simulink library "mpc555extras"  (Simulink 6.0)
settings: Solver=ode45  SolverMode=SingleTasking  StartTime=0.0  StopTime=10.0  RelTol=1e-3
undefined symbols (not defined in the file or in its folder): INT_LEVEL6
libraries: mpc555extras x13, driver_interface_library x7, simulink x4, mpc555interrupts x1
settings Model: Creator=The MathWorks Inc.  LastModifiedBy=batserve  ExtModeAutoUpdateStatusClock=off
settings DataIOCC: SignalLoggingName=logsOut
settings OptimizationCC: BooleanDataType=off
settings DebuggingCC: CheckExecutionContextPreStartOutputMsg=on  CheckExecutionContextRuntimeOutputMsg=on  SolverPrmCheckMsg=none
settings HardwareCC: TargetUnknown=on
settings ModelReferenceCC: UpdateModelReferenceTargets=IfOutOfDate

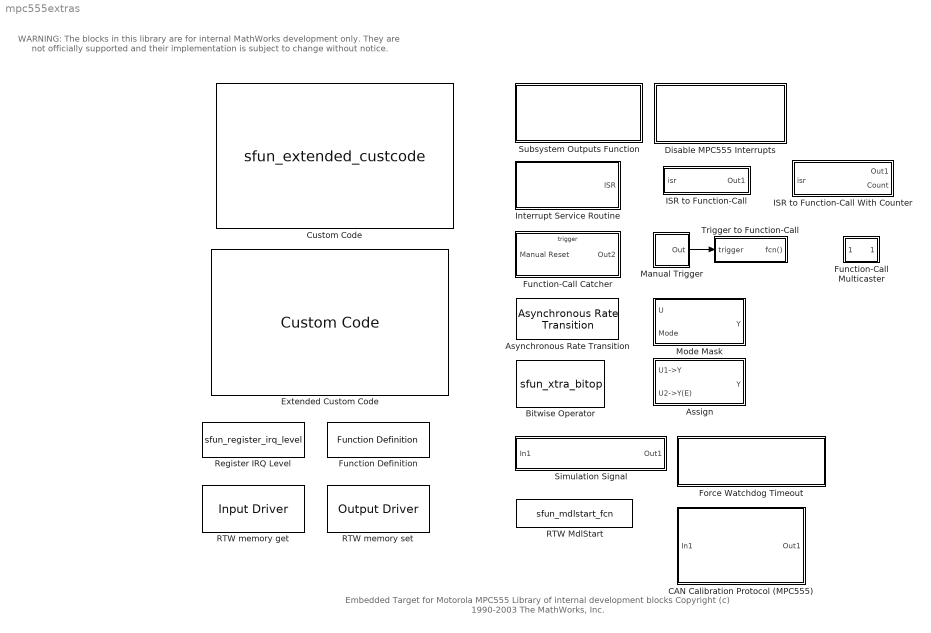
== system mpc555extras ==
  note: WARNING:
      | The blocks in this library are for internal MathWorks development only.
      | They are not officially supported and their implementation is subject to change without notice.
  note: Embedded Target for Motorola MPC555
      | Library of internal development blocks
      | Copyright (c) 1990-2003 The MathWorks, Inc.
  Assign : Subsystem  PropExecContextAcrossSSBoundary=on  mask(Assignment Block){width=5, elements=[2 3]}
      mask prompts: width "Input Width"
      mask help: Replace the specified elements in the input vector with elements from the second vector. You must specify the width of the input signal exactly.
      mask init:
      | elements_split = setdiff([1:width],elements);
      | [s,idx] = sort( [ elements_split elements]);
      | elements_merge = idx;
  Asynchronous Rate Transition : mpc555interrupts/Asynchronous Rate Transition  sample_time=-1
  Bitwise Operator : S-Function  FunctionName=sfun_xtra_bitop  Parameters=UseBitMask,NumInputPorts,BitMask,logicop,zeroTest  mask(Fixed-Point Bitwise Operator){logicop=AND, zeroTest=No Test, UseBitMask=on, NumInputPorts=1, BitMask=bin2dec('11011001'), maskInBinary=off}
      mask prompts: logicop "Operator:"; zeroTest "Zero Test"; UseBitMask "Use bit mask ..."; NumInputPorts "Number of input ports:"; BitMask "Bit Mask"; maskInBinary "Show Mask As Binary"
      mask help: Perform the specified bitwise operation on the inputs. The output data type should represent zero exactly.
      mask init:
      | [BitMask, str ] = sfun_bitop_msk('init',UseBitMask,NumInputPorts,BitMask,logicop,zeroTest);
      mask Help: web(fpbhelp('bitwiseoperator'));
      mask StyleString: popup(AND|OR|NAND|NOR|XOR|NOT|SHIFT LEFT|SHIFT RIGHT|BIT SET|BIT CLEAR|NOT a AND b|a AND NOT b|NOT a OR b|a OR NOT b ),popup(No Test|Test  If Zero|Test If Not Zero),checkbox,edit,edit,checkbox
      mask CallbackString: sfun_bitop_msk('callback')||sfun_bitop_msk('callback')|||
      mask Display: fprintf(['Bitwise\n',str])
  CAN Calibration Protocol (MPC555) : Subsystem  PropExecContextAcrossSSBoundary=on
      mask init:
      | block = 'mpc555drivers/CAN 2.0B Controller Module/CAN Calibration Protocol';                                                                 
      |                                                                           
      | load_system(strtok(block, '/'));                                           
      |                                                                           
      | regexprep(block, '\s',' ');                                                
      | msg = sprintf('Please replace the CCP block with the updated version: "%s" ', block);                             
      | error(msg);
      mask Display: disp(sprintf('Please update\nthe model\nfor a link\nto a\nreplacement block'));
  Custom Code : S-Function  FunctionName=sfun_extended_custcode  mask(Subsystem Custom Coder){unique=Generate for every instance, key='', location=Subsystem Enable Function, top='/* Top Code */', middle='/*Middle Code */', bottom='/*Bottom Code*/'}
      mask prompts: unique "Unique Code Code Generation"
      mask init:
      | [ dispstr,rtwdata ] = mask_custom_code(unique,key,location,top,middle,bottom);
      | set_param(gcb,'rtwdata',rtwdata);
      settings: AttributesFormatString=\n\n
      mask StyleString: popup(Generate for every instance|Generate once per functional mask|Model Singleton),edit,popup(Header File|Parameter File|Source File|Registration File|Subsystem Start Function|Subsystem Initialize Function|Subsystem Terminate Function|Subsystem Enable Function|Subsystem Disable Function|Subsystem Outputs Function|Subsystem Update Function|Subsystem Derivatives Function|Registration Function|Model Start Function|Model Initialize Function|Model Terminate Function|Model Outputs Function|Model Update Function|Model Derivatives Function),edit,edit,edit
      mask Display: text(0.1,0.5,dispstr,'horizontalAlignment','left')
  Disable MPC555 Interrupts : Subsystem  Tag=Disable MPC555 Interrupts  PropExecContextAcrossSSBoundary=on  mask(Disable MPC555 Interrupts){}
      mask help:
      | Disable MPC555 Interrupts during the model outputs function.
      |
      | Be carefull using this block as it may block a faster rate task from executing in time. Use it only in atomic subsystems that may be accessing hardware resources that need protection against interrupt access.
      mask init:
      | [top,bottom,dispstr] = mpc555_disable_interrupts('getcode',gcb);
      mask Display: disp(dispstr)
  Extended Custom Code : driver_interface_library/Custom Code
  Force Watchdog Timeout : Subsystem  TreatAsAtomicUnit=on  PropExecContextAcrossSSBoundary=on  mask(Processor Reset){}
      mask help:
      | As soon as this block executes interrupts are disabled and the processor enters an infinite loop. The watchdog timer will then time out and reset the processor.
      |
      | This block mus be placed in an action subsystem such as an if, then, else subsystem or a function call subsystem.
      mask init:
      | read_tunable_parameters;
      mask Help:
      | As soon as this block executes interrupts are disabled and the processor enters an infinite loop. The watchdog timer will then time out and reset the processor.<p>
      | 
      | This block mus be placed in an action subsystem such as an if, then, else subsystem or a function call subsystem.
      mask Display: disp('Processor Reset\nForce Watchdog Timeout');
  Function Definition : driver_interface_library/Function Definition  function_name='void func(void)'
  Function-Call Multicaster : Subsystem  PropExecContextAcrossSSBoundary=on
      mask Type: Function Call Multicaster
      mask Description: The input to this block should be a function call. The output of the block can be demuxed so that multiple function call subsystems can be triggered off the same function call.
      mask Display:
      | plot([0 2],[0.5 0.5]);
      | plot([0.5 1],[0.6 0.6]);
      | plot([0.5 1],[0.4 0.4]);
      | plot([0.8 1],[0.7 0.7]);
      | plot([0.8 1],[0.3 0.3]);
      | 
      | plot([1 1],[0.3 0.7])
      | plot([0.95 0.95],[0.2 0.8])
      | plot([0.9 0.9],[0.2 0.8])
  Function-Call Catcher : Subsystem  TreatAsAtomicUnit=on  PropExecContextAcrossSSBoundary=on
      mask Type: Function Call Catcher
      mask Description: Feed in multiple function call trigger via a mux into the top. The block wait till every function trigger has fired at least once before firing it's output trigger then reseting it's counters
  ISR to Function-Call : Subsystem  PropExecContextAcrossSSBoundary=on  mask{t=1}
      mask prompts: t "Sample Period"
      mask help: Converts an interrupt service routine call to a "if action" call at a specified sample rate.
      settings: AttributesFormatString=sample time = %<t>
      mask Display:
      | plot([0.2 0.4 0.5 0.6 0.7 0.75 ],[0.5 0.5 0.7 0.3 0.5 0.5])
      | plot([0.2 0.4 0.5 0.6 0.7 0.75 ],1-[0.5 0.5 0.7 0.3 0.5 0.5])
      | plot([0.2 0.4 0.5 0.6 0.7 0.75 ],1- [0.5 0.5 0.7 0.3 0.5 0.5]+0.1)
      | port_label('input',1,'isr')
      | port_label('output',1,'if { }')
  ISR to Function-Call With Counter : Subsystem  PropExecContextAcrossSSBoundary=on  mask{t=1}
      mask prompts: t "Sample Period"
      mask help: Converts an interrupt service routine call to a "if action" call at a specified sample rate. It also has an output that provides the number of times the interrupt has executed since it was last polled.
      settings: AttributesFormatString=sample time = %<t>
      mask Display:
      | plot([0.2 0.4 0.5 0.6 0.7 0.75 ],[0.5 0.5 0.7 0.3 0.5 0.5])
      | plot([0.2 0.4 0.5 0.6 0.7 0.75 ],1-[0.5 0.5 0.7 0.3 0.5 0.5])
      | plot([0.2 0.4 0.5 0.6 0.7 0.75 ],1- [0.5 0.5 0.7 0.3 0.5 0.5]+0.1)
      | port_label('input',1,'isr')
      | port_label('output',1,'if { }')
      | port_label('output',2,'count')
  Interrupt Service Routine : Subsystem  PropExecContextAcrossSSBoundary=on  mask{callback=EXT_IRQ0, float_flag=Yes}
      mask prompts: callback "ISR Source"; float_flag "Uses Floating Point?"
      mask help: Choose the interrupt source for your ISR generator. For faster interrupts you can choose not to support floating point. However if you choose not to support floating point in the system and you place blocks in the system that do you floating point operation then the program will throw a floating point exception at run-time.
      mask init:
      | [f_proto,dispstr,reg_callback ]  = mask_isr_callback(gcbh,callback,float_flag);
      mask StyleString: popup(EXT_IRQ0|INT_LEVEL0|EXT_IRQ1|INT_LEVEL1|EXT_IRQ2|INT_LEVEL2|EXT_IRQ3|INT_LEVEL3|EXT_IRQ4|INT_LEVEL4|EXT_IRQ5|INT_LEVEL5|EXT_IRQ6|INT_LEVEL6|EXT_IRQ7|INT_LEVEL7|INT_LEVEL8|INT_LEVEL9|INT_LEVEL10|INT_LEVEL11|INT_LEVEL12|INT_LEVEL13|INT_LEVEL14|INT_LEVEL15|INT_LEVEL16|INT_LEVEL17|INT_LEVEL18|INT_LEVEL19|INT_LEVEL20|INT_LEVEL21|INT_LEVEL22|INT_LEVEL23|INT_LEVEL24|INT_LEVEL25|INT_LEVEL26|INT_LEVEL27|INT_LEVEL28|INT_LEVEL29|INT_LEVEL30|INT_LEVEL31),popup(Yes|No)
      mask Display: disp(dispstr)
  Manual Trigger : Subsystem  PropExecContextAcrossSSBoundary=on  mask(Manual Trigger){value=-1}
      mask prompts: value "Output value:"
      mask init:
      | if (value==1)
      |   dispStr = 'HIGH';
      | else % (value == -1)
      |   dispStr = 'LOW';
      | end
      settings: OpenFcn=oldValue = str2num(get_param(gcb, 'value')); if (oldValue==1), set_param(gcb, 'value', '-1'); else, set_param(gcb, 'value', '1'); end
      mask Display: disp(dispStr)
  Mode Mask : Subsystem  PropExecContextAcrossSSBoundary=on  mask(Mode based mask){width=5, elements=[2 3], mode_inputs=[1 2], mode_outputs=[0 0]}
      mask prompts: width "Input Width"; elements "Mode Elements"; mode_inputs "Mode Inputs"; mode_outputs "Mode Outputs"
      mask help: Enables selective switching of input elements based on a single scalar mode value.
      mask Help:
      | <ul>
      | <li>Specify the input width exactly.
      | <li>The mode elements are the elements of the input
      | vector that can be switched. Specify their indicies
      | <li> The mode inputs are the mode values for each input
      | that when the mode input equals the value the input element
      | will be switched
      | <li> The mode outputs are the alternative values for each element that is switched in if it's mode value is equal.
      | </ul>
  RTW MdlStart : S-Function  FunctionName=sfun_mdlstart_fcn
      mask Type: RTW MdlStart Function
      mask Description:
      | Forces downstream triggered blocks to run at mdlStart.
      | 
      | Be carefull with this block. You should not put in the triggered subsystem any blocks
      | which have state. This block is primarily to be used to perform device driver initialization.
      | 
      | The blocks in the downstream triggered subsystem will not run during simulation
      | or Simulink Accelerator.
      mask Display: disp('RTW MdlStart Function')
  RTW memory get : driver_interface_library/Input Driver  t=1  expr='MIOS1[%<i>][%<p>]'  portWidth=6  pOpt=[2 3 6 8 3 9]  expression_type=Not expression
  RTW memory set : driver_interface_library/Output Driver  operation_type=LHS Assignment  input_is_contiguous=off  t=-1  expr='*Y_ADDR'  port_width=1  pOpt=[]
  Register IRQ Level : S-Function  FunctionName=sfun_register_irq_level  Parameters=irqLevel  mask{irqLevel=INT_LEVEL6}
      mask prompts: irqLevel "IRQ Level"
      mask Display: disp('Register IRQ level')
  Simulation Signal : Subsystem  PropExecContextAcrossSSBoundary=on  mask(Simulation-only signal){baseName=SimSignal}
      mask prompts: baseName "Base name for signal identifier:"
      mask help: Only produce an identifier for this signal when generating code for use in simulation (e.g., Accelerator, Processor-in-the-loop and S-Function targets).
      mask init:
      | InportBlock = [gcb, '/In1'];
      | hPorts = get_param(InportBlock, 'PortHandles');
      | hPort = hPorts.Outport;
      | signalName = getuniquesignalname(hPort, baseName);
      | eval([signalName, '=SimOnly.Signal;']);
      | set_param(hPort, 'Name', signalName);
      mask Display: disp(['SimOnlySignal: ', signalName])
  Subsystem Outputs Function : Subsystem  PropExecContextAcrossSSBoundary=on
      settings: OpenFcn=ccopenfcn('Subsystem Outputs Function')
      mask Type: Subsystem Outputs Function
      mask Description: Place this block in an atomic subsystem to ensure that the subsystem is protected from interrupts during the model outputs function. This block should not be used recursively.
      mask Display: disp('Disable Interrupts \nIn Outputs Function Of\nAtomic Subsytem');
  Trigger to Function-Call : Subsystem  PropExecContextAcrossSSBoundary=on
      mask Type: Trigger to function call conversion
      mask Description: Converts a Simulink trigger signal to a function call trigger signal.
  wires:
  Manual Trigger/1(Out) -> Trigger to Function-Call/1(trigger)

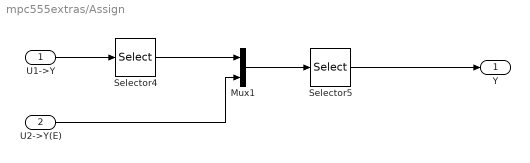
== system mpc555extras/Assign ==
  U1->Y : Inport  Port=1  LatchInput=off
  U2->Y(E) : Inport  Port=2  LatchInput=off
  Mux1 : Mux  Inputs=2
  Selector4 : Selector  Elements=elements_split  InputPortWidth=width
  Selector5 : Selector  Elements=elements_merge  InputPortWidth=width
  Y : Outport
  wires:
  Selector4/1 -> Mux1/1
  Mux1/1 -> Selector5/1
  U1->Y/1 -> Selector4/1
  Selector5/1 -> Y/1
  U2->Y(E)/1 -> Mux1/2

== system mpc555extras/CAN Calibration Protocol (MPC555) ==
  In1 : Inport  Port=1  LatchInput=off
  Out1 : Outport
  wires:
  In1/1 -> Out1/1

== system mpc555extras/Disable MPC555 Interrupts ==
  Disable MPC555 Interrupts : mpc555extras/Custom Code  Tag=Disable MPC555 Interrupts  unique=Generate for every instance  key=''  location=Subsystem Outputs Function  top=top  middle=''  bottom=bottom

== system mpc555extras/Force Watchdog Timeout ==
  Constant : Constant
  Force Watchdog Timeout : mpc555extras/Custom Code  unique=Generate for every instance  key=''  location=Subsystem Outputs Function  top=''  middle=''  bottom='EID(); for(;;);'
  Terminator : Terminator
  wires:
  Constant/1 -> Terminator/1

== system mpc555extras/Function-Call Multicaster ==
  fcn_in : Inport  Port=1  LatchInput=off
  Subsystem : Subsystem  TreatAsAtomicUnit=on  PropExecContextAcrossSSBoundary=on
  fcn1 : Outport
  wires:
  Subsystem/1(Out1) -> fcn1/1
  fcn_in/1 -> Subsystem/Trigger

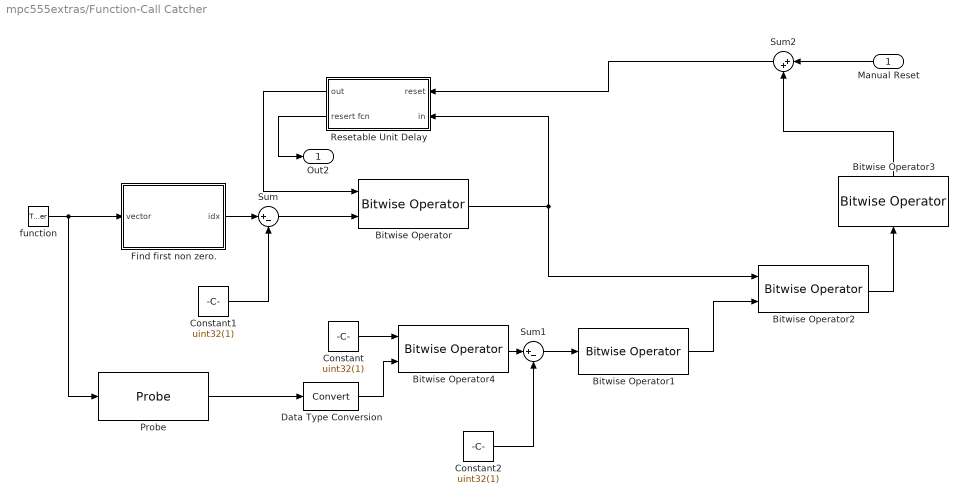
== system mpc555extras/Function-Call Catcher ==
  Manual Reset : Inport  Orientation=left  Port=1  LatchInput=off
  function : TriggerPort  TriggerType=function-call  StatesWhenEnabling=reset  ShowOutputPort=on  OutputDataType=int8  ZeroCross=off
  Bitwise Operator : mpc555extras/Bitwise Operator  logicop=BIT SET  zeroTest=No Test  UseBitMask=off  NumInputPorts=2  BitMask=bin2dec('11011001')  maskInBinary=off
  Bitwise Operator1 : mpc555extras/Bitwise Operator  logicop=NOT  zeroTest=No Test  UseBitMask=on  BitMask=bin2dec('11011001')  maskInBinary=off
  Bitwise Operator2 : mpc555extras/Bitwise Operator  logicop=OR  zeroTest=No Test  UseBitMask=off  NumInputPorts=2  BitMask=bin2dec('11011001')  maskInBinary=off
  Bitwise Operator3 : mpc555extras/Bitwise Operator  Orientation=up  logicop=NOT  zeroTest="Test  If Zero"  UseBitMask=on  BitMask=bin2dec('11011001')  maskInBinary=off
  Bitwise Operator4 : mpc555extras/Bitwise Operator  logicop=SHIFT LEFT  zeroTest=No Test  UseBitMask=off  NumInputPorts=2  BitMask=bin2dec('11011001')  maskInBinary=off
  Constant : Constant  Value=uint32(1)
  Constant1 : Constant  Value=uint32(1)
  Constant2 : Constant  Value=uint32(1)
  Data Type Conversion : DataTypeConversion  OutDataTypeMode=uint32  RndMeth=Zero
  Find first non zero. : Subsystem  PropExecContextAcrossSSBoundary=on
  Probe : Probe  ProbeSampleTime=off  ProbeComplexSignal=off
  Resetable Unit Delay : Subsystem  Orientation=left  PropExecContextAcrossSSBoundary=on  mask(Resetable Unit Delay){reset=uint32(0), t=-1}
      mask prompts: reset "Initial State"; t "Sample Time"
  Sum : Sum  Inputs=|+-  InputSameDT=on
  Sum1 : Sum  Inputs=|+-  InputSameDT=on
  Sum2 : Sum  Orientation=left  Inputs=|++  SaturateOnIntegerOverflow=on  InputSameDT=on
  Out2 : Outport
  wires:
  Sum2/1 -> Resetable Unit Delay/1(reset)
  Bitwise Operator3/1 -> Sum2/2
  Manual Reset/1 -> Sum2/1
  Constant2/1 -> Sum1/2
  Sum1/1 -> Bitwise Operator1/1
  Bitwise Operator4/1 -> Sum1/1
  Constant/1 -> Bitwise Operator4/1
  Bitwise Operator2/1 -> Bitwise Operator3/1
  Bitwise Operator1/1 -> Bitwise Operator2/2
  Resetable Unit Delay/1(out) -> Bitwise Operator/1
  Bitwise Operator/1 -> Bitwise Operator2/1, Resetable Unit Delay/2(in)
  function/1 -> Probe/1, Find first non zero./1(vector)
  Find first non zero./1(idx) -> Sum/1
  Sum/1 -> Bitwise Operator/2
  Constant1/1 -> Sum/2
  Resetable Unit Delay/2(resert fcn) -> Out2/1
  Data Type Conversion/1 -> Bitwise Operator4/2
  Probe/1 -> Data Type Conversion/1

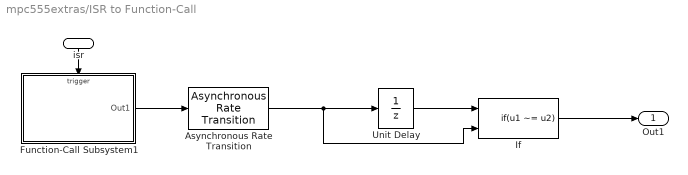
== system mpc555extras/ISR to Function-Call ==
  isr : Inport  Orientation=down  Port=1  LatchInput=off
  Asynchronous Rate Transition : mpc555extras/Asynchronous Rate Transition  sample_time=-1
  Function-Call Subsystem1 : Subsystem  TreatAsAtomicUnit=on  PropExecContextAcrossSSBoundary=on
  If : If  NumInputs=2  IfExpression=u1 ~= u2  ShowElse=off  ZeroCross=off
  Unit Delay : UnitDelay  SampleTime=t
  Out1 : Outport
  wires:
  Function-Call Subsystem1/1(Out1) -> Asynchronous Rate Transition/1
  Asynchronous Rate Transition/1 -> If/2, Unit Delay/1
  isr/1 -> Function-Call Subsystem1/Trigger
  If/1 -> Out1/1
  Unit Delay/1 -> If/1

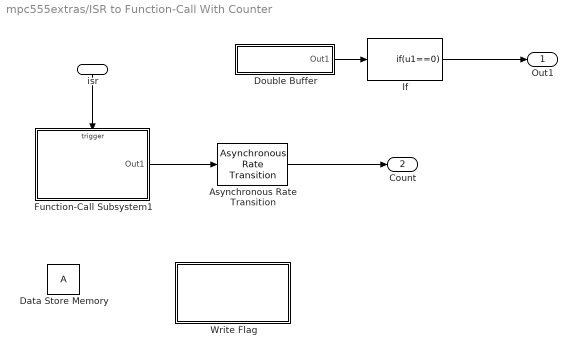
== system mpc555extras/ISR to Function-Call With Counter ==
  isr : Inport  Orientation=down  Port=1  LatchInput=off
  Asynchronous Rate Transition : mpc555extras/Asynchronous Rate Transition  sample_time=t
  Data Store Memory : DataStoreMemory  DialogController=Simulink.DDGSource  DataStoreName=A  InitialValue=1
  Double Buffer : Subsystem  TreatAsAtomicUnit=on  PropExecContextAcrossSSBoundary=on
  Function-Call Subsystem1 : Subsystem  TreatAsAtomicUnit=on  PropExecContextAcrossSSBoundary=on
  If : If  IfExpression=u1==0  ShowElse=off  ZeroCross=off
  Write Flag : Subsystem  TreatAsAtomicUnit=on  PropExecContextAcrossSSBoundary=on
  Out1 : Outport
  Count : Outport  Port=2
  wires:
  Double Buffer/1(Out1) -> If/1
  Asynchronous Rate Transition/1 -> Count/1
  If/1 -> Out1/1
  isr/1 -> Function-Call Subsystem1/Trigger
  Function-Call Subsystem1/1(Out1) -> Asynchronous Rate Transition/1

== system mpc555extras/Interrupt Service Routine ==
  Custom Code : mpc555extras/Custom Code  unique=Generate for every instance  key=''  location=Model Start Function  top=reg_callback  middle=''  bottom=''
  Function Definition : driver_interface_library/Function Definition  function_name=f_proto
  Header File : Subsystem  Tag=line1 line2  PropExecContextAcrossSSBoundary=on
      settings: CopyFcn=cccopyfcn(gcb)  OpenFcn=ccopenfcn('Header File')
      mask Type: Header File
      mask Description: Add code to model .h file
      mask Help: This header file block contains text fields to insert custom user code at the top and bottom of model.h file.
      mask Display: disp('Header\nFile');
  ISR : Outport
  wires:
  Function Definition/1 -> ISR/1

== system mpc555extras/Manual Trigger ==
  Output value : Constant  Value=value
  Out : Outport
  wires:
  Output value/1 -> Out/1

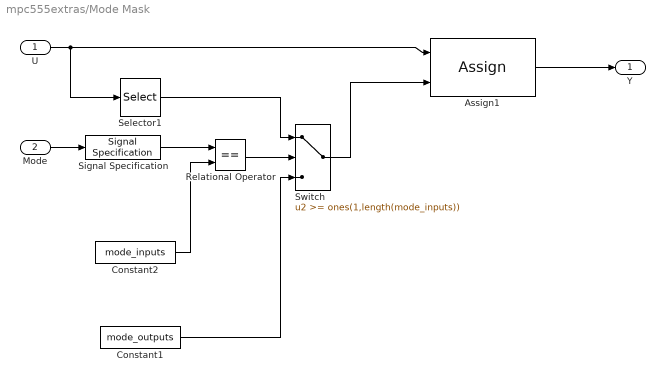
== system mpc555extras/Mode Mask ==
  U : Inport  Port=1  LatchInput=off
  Mode : Inport  Port=2  LatchInput=off
  Assign1 : mpc555extras/Assign  width=width  elements=elements
  Constant1 : Constant  Value=mode_outputs
  Constant2 : Constant  Value=mode_inputs
  Relational Operator : RelationalOperator  Operator===  InputSameDT=on
  Selector1 : Selector  Elements=elements  InputPortWidth=width
  Signal Specification : simulink/Signal Attributes/Signal Specification  D=1  Ts=-1  DataType=auto  OutDataType=sfix(16)  OutScaling=2^0
      settings: SignalType=auto  SamplingMode=auto
  Switch : Switch  Threshold=ones(1,length(mode_inputs))  InputSameDT=on
  Y : Outport
  wires:
  Constant2/1 -> Relational Operator/2
  Relational Operator/1 -> Switch/2
  U/1 -> Assign1/1, Selector1/1
  Constant1/1 -> Switch/3
  Selector1/1 -> Switch/1
  Switch/1 -> Assign1/2
  Assign1/1 -> Y/1
  Mode/1 -> Signal Specification/1
  Signal Specification/1 -> Relational Operator/1

== system mpc555extras/Simulation Signal ==
  In1 : Inport  Port=1  LatchInput=off
  Out1 : Outport
  wires:
  In1/1 -> Out1/1  "SimSignal1"

== system mpc555extras/Subsystem Outputs Function ==

== system mpc555extras/Trigger to Function-Call ==
  trigger : Inport  Orientation=down  Port=1  LatchInput=off
  trigger2fcn : Subsystem  TreatAsAtomicUnit=on  PropExecContextAcrossSSBoundary=on
  fcn() : Outport
  wires:
  trigger2fcn/1(fcn()) -> fcn()/1
  trigger/1 -> trigger2fcn/Trigger

== system mpc555extras/Function-Call Multicaster/Subsystem ==
  Trigger : TriggerPort  TriggerType=function-call  StatesWhenEnabling=reset  ZeroCross=off
  Function-Call Generator : simulink/Ports & Subsystems/Function-Call Generator  sample_time=-1  numberOfIterations=1
  Out1 : Outport
  wires:
  Function-Call Generator/1 -> Out1/1

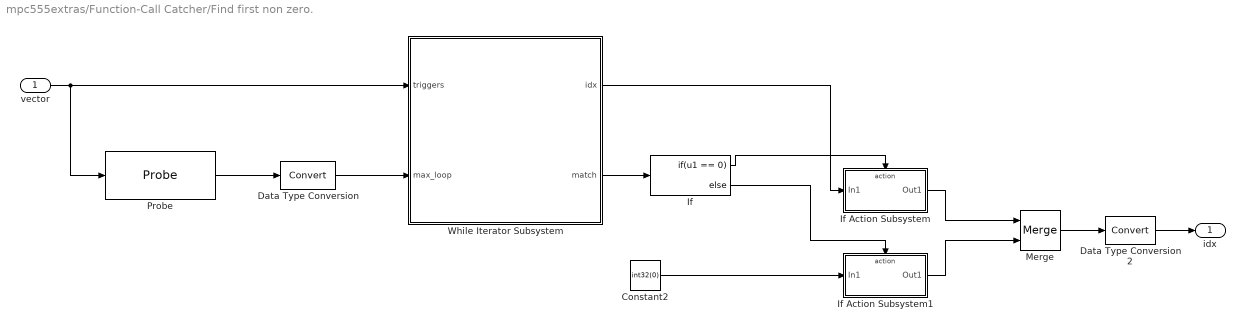
== system mpc555extras/Function-Call Catcher/Find first non zero. ==
  vector : Inport  Port=1  LatchInput=off
  Constant2 : Constant  Value=int32(0)
  Data Type Conversion : DataTypeConversion  OutDataTypeMode=int32  RndMeth=Zero
  Data Type Conversion2 : DataTypeConversion  OutDataTypeMode=uint32  RndMeth=Zero
  If : If  IfExpression=u1 == 0  ZeroCross=off
  If Action Subsystem : Subsystem  TreatAsAtomicUnit=on  PropExecContextAcrossSSBoundary=on
  If Action Subsystem1 : Subsystem  TreatAsAtomicUnit=on  PropExecContextAcrossSSBoundary=on
  Merge : Merge
  Probe : Probe  ProbeSampleTime=off  ProbeComplexSignal=off
  While Iterator Subsystem : Subsystem  TreatAsAtomicUnit=on  PropExecContextAcrossSSBoundary=on
  idx : Outport
  wires:
  Data Type Conversion/1 -> While Iterator Subsystem/2(max_loop)
  Merge/1 -> Data Type Conversion2/1
  If Action Subsystem1/1(Out1) -> Merge/2
  If Action Subsystem/1(Out1) -> Merge/1
  If/2 -> If Action Subsystem1/Action
  If/1 -> If Action Subsystem/Action
  Constant2/1 -> If Action Subsystem1/1(In1)
  While Iterator Subsystem/2(match) -> If/1
  While Iterator Subsystem/1(idx) -> If Action Subsystem/1(In1)
  Probe/1 -> Data Type Conversion/1
  vector/1 -> While Iterator Subsystem/1(triggers), Probe/1
  Data Type Conversion2/1 -> idx/1

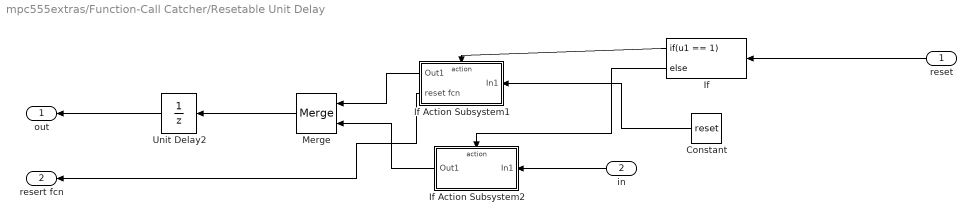
== system mpc555extras/Function-Call Catcher/Resetable Unit Delay ==
  reset : Inport  Orientation=left  Port=1  LatchInput=off
  in : Inport  Orientation=left  Port=2  LatchInput=off
  Constant : Constant  Orientation=left  Value=reset
  If : If  Orientation=left  IfExpression=u1 == 1  ZeroCross=off
  If Action Subsystem1 : Subsystem  Orientation=left  TreatAsAtomicUnit=on  PropExecContextAcrossSSBoundary=on
  If Action Subsystem2 : Subsystem  Orientation=left  TreatAsAtomicUnit=on  PropExecContextAcrossSSBoundary=on
  Merge : Merge  Orientation=left
  Unit Delay2 : UnitDelay  Orientation=left  X0=reset  SampleTime=t
  out : Outport  Orientation=left
  resert fcn : Outport  Orientation=left  Port=2
  wires:
  in/1 -> If Action Subsystem2/1(In1)
  Merge/1 -> Unit Delay2/1
  reset/1 -> If/1
  If Action Subsystem1/1(Out1) -> Merge/1
  If Action Subsystem2/1(Out1) -> Merge/2
  Constant/1 -> If Action Subsystem1/1(In1)
  If/2 -> If Action Subsystem2/Action
  If/1 -> If Action Subsystem1/Action
  Unit Delay2/1 -> out/1
  If Action Subsystem1/2(reset fcn) -> resert fcn/1

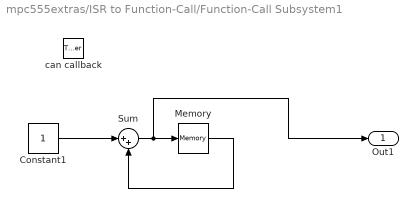
== system mpc555extras/ISR to Function-Call/Function-Call Subsystem1 ==
  can callback : TriggerPort  TriggerType=function-call  StatesWhenEnabling=reset  ZeroCross=off
  Constant1 : Constant
  Memory : Memory  X0=1  InheritSampleTime=on
  Sum : Sum  Inputs=|++  InputSameDT=on
  Out1 : Outport  InitialOutput=0
  wires:
  Constant1/1 -> Sum/1
  Sum/1 -> Memory/1, Out1/1
  Memory/1 -> Sum/2

== system mpc555extras/ISR to Function-Call With Counter/Double Buffer ==
  Custom Code : mpc555extras/Custom Code  unique=Generate for every instance  key=''  location=Subsystem Outputs Function  top='EID();'  middle=''  bottom='EIE();'
  Data Store Read : DataStoreRead  DialogController=Simulink.DDGSource  DataStoreName=A  SampleTime=t
  Out1 : Outport
  wires:
  Data Store Read/1 -> Out1/1

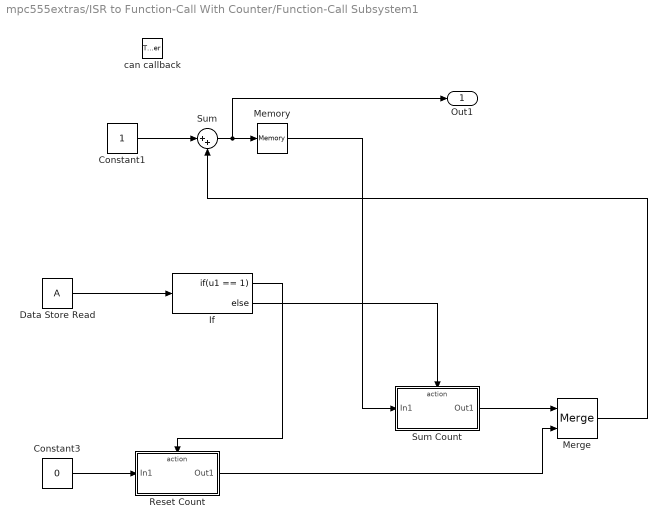
== system mpc555extras/ISR to Function-Call With Counter/Function-Call Subsystem1 ==
  can callback : TriggerPort  TriggerType=function-call  StatesWhenEnabling=reset  ZeroCross=off
  Constant1 : Constant
  Constant3 : Constant  Value=0
  Data Store Read : DataStoreRead  DialogController=Simulink.DDGSource  DataStoreName=A  SampleTime=-1
  If : If  IfExpression=u1 == 1  ZeroCross=off
  Memory : Memory  X0=1  InheritSampleTime=on
  Merge : Merge
  Reset Count : Subsystem  TreatAsAtomicUnit=on  PropExecContextAcrossSSBoundary=on
  Sum : Sum  Inputs=|++  InputSameDT=on
  Sum Count : Subsystem  TreatAsAtomicUnit=on  PropExecContextAcrossSSBoundary=on
  Out1 : Outport  InitialOutput=0
  wires:
  If/1 -> Reset Count/Action
  If/2 -> Sum Count/Action
  Data Store Read/1 -> If/1
  Merge/1 -> Sum/2
  Sum Count/1(Out1) -> Merge/1
  Reset Count/1(Out1) -> Merge/2
  Memory/1 -> Sum Count/1(In1)
  Constant3/1 -> Reset Count/1(In1)
  Sum/1 -> Out1/1, Memory/1
  Constant1/1 -> Sum/1

== system mpc555extras/ISR to Function-Call With Counter/Write Flag ==
  Custom Code : mpc555extras/Custom Code  unique=Generate for every instance  key=''  location=Subsystem Outputs Function  top='EID();'  middle=''  bottom='EIE();'
  Data Store Write : DataStoreWrite  DialogController=Simulink.DDGSource  DataStoreName=A  SampleTime=-1
  RTW memory get : driver_interface_library/Input Driver  t=t  expr=1  portWidth=6  pOpt=[2 3 6 8 3 9]  expression_type=Not expression
  wires:
  RTW memory get/1 -> Data Store Write/1

== system mpc555extras/Interrupt Service Routine/Header File ==

== system mpc555extras/Trigger to Function-Call/trigger2fcn ==
  Trigger : TriggerPort  TriggerType=either  StatesWhenEnabling=reset  ZeroCross=off
  Function-Call Generator : simulink/Ports & Subsystems/Function-Call Generator  sample_time=-1  numberOfIterations=1
  fcn() : Outport
  wires:
  Function-Call Generator/1 -> fcn()/1

== system mpc555extras/Function-Call Catcher/Find first non zero./If Action Subsystem ==
  In1 : Inport  Port=1  LatchInput=off
  Action Port : ActionPort
  Out1 : Outport
  wires:
  In1/1 -> Out1/1

== system mpc555extras/Function-Call Catcher/Find first non zero./If Action Subsystem1 ==
  In1 : Inport  Port=1  LatchInput=off
  Action Port : ActionPort
  Out1 : Outport
  wires:
  In1/1 -> Out1/1

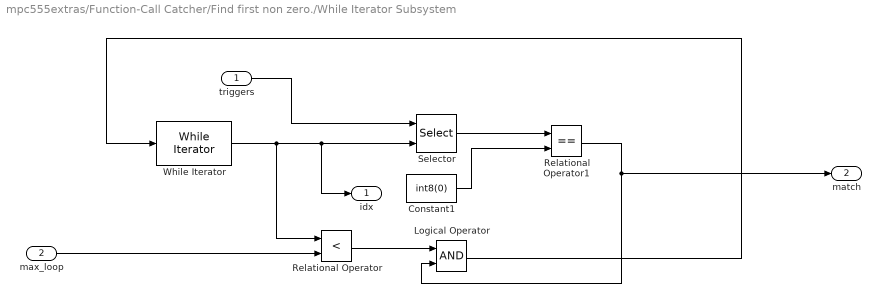
== system mpc555extras/Function-Call Catcher/Find first non zero./While Iterator Subsystem ==
  triggers : Inport  Port=1  LatchInput=off
  max_loop : Inport  Port=2  DataType=int32  LatchInput=off
  Constant1 : Constant  Value=int8(0)
  Logical Operator : Logic
  Relational Operator : RelationalOperator  Operator=<  InputSameDT=on
  Relational Operator1 : RelationalOperator  Operator===  InputSameDT=on
  Selector : Selector  ElementSrc=External  Elements=[1 3]
  While Iterator : WhileIterator  MaxIters=-1  WhileBlockType=do-while  ResetStates=reset  ShowIterationPort=on
  idx : Outport
  match : Outport  Port=2
  wires:
  triggers/1 -> Selector/1
  While Iterator/1 -> Relational Operator/1, Selector/2, idx/1
  max_loop/1 -> Relational Operator/2
  Relational Operator/1 -> Logical Operator/1
  Selector/1 -> Relational Operator1/1
  Constant1/1 -> Relational Operator1/2
  Relational Operator1/1 -> match/1, Logical Operator/2
  Logical Operator/1 -> While Iterator/1

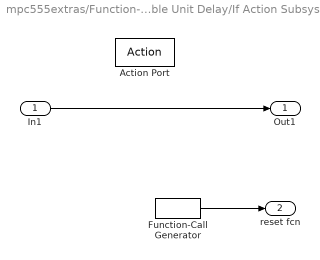
== system mpc555extras/Function-Call Catcher/Resetable Unit Delay/If Action Subsystem1 ==
  In1 : Inport  Port=1  LatchInput=off
  Action Port : ActionPort
  Function-Call Generator : simulink/Ports & Subsystems/Function-Call Generator  sample_time=-1  numberOfIterations=1
  Out1 : Outport
  reset fcn : Outport  Port=2
  wires:
  In1/1 -> Out1/1
  Function-Call Generator/1 -> reset fcn/1

== system mpc555extras/Function-Call Catcher/Resetable Unit Delay/If Action Subsystem2 ==
  In1 : Inport  Port=1  LatchInput=off
  Action Port : ActionPort
  Out1 : Outport
  wires:
  In1/1 -> Out1/1

== system mpc555extras/ISR to Function-Call With Counter/Function-Call Subsystem1/Reset Count ==
  In1 : Inport  Port=1  LatchInput=off
  Action Port : ActionPort
  Data Store Write : DataStoreWrite  DialogController=Simulink.DDGSource  DataStoreName=A  SampleTime=-1
  RTW memory get : driver_interface_library/Input Driver  t=-1  expr=0  portWidth=6  pOpt=[2 3 6 8 3 9]  expression_type=Not expression
  Out1 : Outport
  wires:
  RTW memory get/1 -> Data Store Write/1
  In1/1 -> Out1/1

== system mpc555extras/ISR to Function-Call With Counter/Function-Call Subsystem1/Sum Count ==
  In1 : Inport  Port=1  LatchInput=off
  Action Port : ActionPort
  Out1 : Outport
  wires:
  In1/1 -> Out1/1
